simulink model "four_channel_bilateral_teleoperation_architecture_discrete"  (R2021a)
settings: Solver=FixedStepAuto  StartTime=0.0  StopTime=4.0  FixedStep=0.001  RelTol=1e-3
values from neighbouring files (symbols this model uses):
  A = 1    [four_channel_bilateral_teleoperation_architecture_params.m]
  Be = 0    [four_channel_bilateral_teleoperation_architecture_params.m]    (also in params_teleop.m = 100)
  Bh = 70    [four_channel_bilateral_teleoperation_architecture_params.m]    (also in params_teleop.m)
  Bm = 0.8    [four_channel_bilateral_teleoperation_architecture_params.m]    (also in params_teleop.m)
  Bs = 0.8*4    (= 3.2)    [four_channel_bilateral_teleoperation_architecture_params.m]    (also in params_teleop.m)
  Dh = 1000    [four_channel_bilateral_teleoperation_architecture_params.m]
  Dm = 0    [four_channel_bilateral_teleoperation_architecture_params.m]    (also in params_teleop.m)
  Ds = 0    [four_channel_bilateral_teleoperation_architecture_params.m]    (also in params_teleop.m)
  Fc = 1    [four_channel_bilateral_teleoperation_architecture_params.m]
  Fip = 1    [four_channel_bilateral_teleoperation_architecture_params.m]
  Je = 0    [four_channel_bilateral_teleoperation_architecture_params.m]    (also in params_teleop.m)
  Jh = 0.5    [four_channel_bilateral_teleoperation_architecture_params.m]    (also in params_teleop.m)
  Ke = 200    [four_channel_bilateral_teleoperation_architecture_params.m]    (also in params_teleop.m)
  Kh = 2000    [four_channel_bilateral_teleoperation_architecture_params.m]    (also in params_teleop.m)
  Km = 1    [four_channel_bilateral_teleoperation_architecture_params.m]    (also in params_teleop.m)
  Ks = 4    [four_channel_bilateral_teleoperation_architecture_params.m]    (also in params_teleop.m)
  Mm = 0.5    [four_channel_bilateral_teleoperation_architecture_params.m]    (also in params_teleop.m)
  Ms = 2    [four_channel_bilateral_teleoperation_architecture_params.m]    (also in params_teleop.m)
  Ph = 20000    [four_channel_bilateral_teleoperation_architecture_params.m]
  tau = 10000    [four_channel_bilateral_teleoperation_architecture_params.m]
  Ts = 0.001    [four_channel_bilateral_teleoperation_architecture_params.m]
libraries: simulink x7
settings Model: Creator=anuj  LastModifiedBy=antoninoparisi
settings SolverCC: AlgebraicLoopSolver=TrustRegion
settings DebuggingCC: SFMachineParentedDataDiag=warning

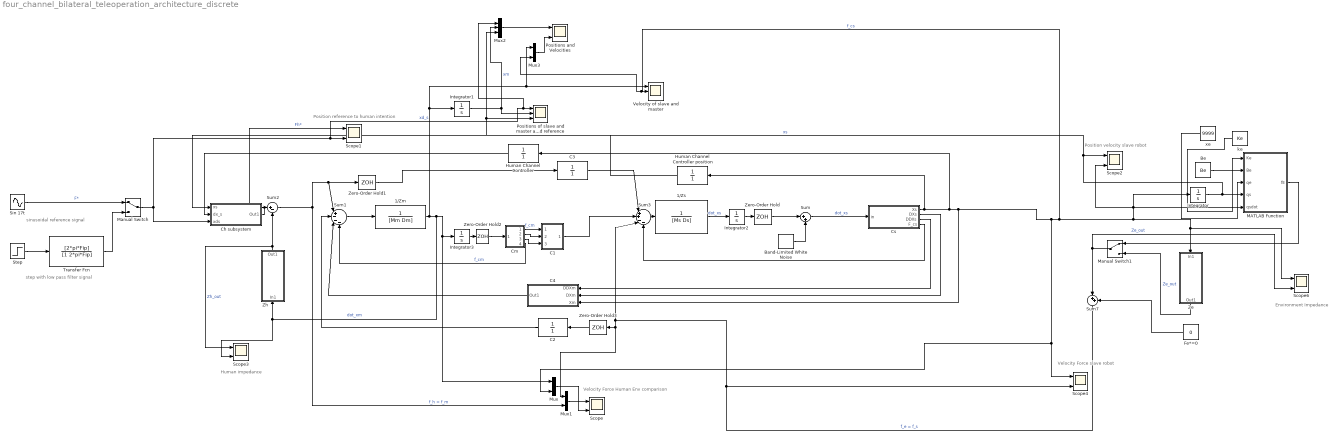
== system four_channel_bilateral_teleoperation_architecture_discrete ==
  note: Environment Impedance
  note: Human impedance
  note: Velocity Force Human Env comparison
  note: Velocity Force slave robot
  note: Position velocity slave robot
  note: sinusoidal reference signal
  note: step with low pass filter signal
  note: Position reference to human intention
  1/Zm : TransferFcn  Denominator=[Mm Dm]
  1/Zs : TransferFcn  Denominator=[Ms Ds]
  Band-Limited White Noise : simulink/Sources/Band-Limited White Noise  Cov=[0.000001]  Ts=Ts  seed=[23341]
  Be : Constant  Value=Be
  C1 : Subsystem
  C2 : TransferFcn  Denominator=[1]
  C3 : TransferFcn  Denominator=[1]
  C4 : Subsystem
  Ch subsystem : Subsystem
  Cm : Subsystem
  Cs : Subsystem
  Fe*=0 : Constant  Value=0
  Human Channel Controller : TransferFcn  Denominator=[1]
  Human Channel Controller position : TransferFcn  Denominator=[1]
  Integrator{,1..3} (4 alike) : Integrator
  MATLAB Function : MATLAB Function  TreatAsAtomicUnit=on
  Manual Switch : ManualSwitch
  Manual Switch1 : ManualSwitch
  Mux : Mux  Inputs=2
  Mux1 : Mux  Inputs=2
  Mux2 : Mux  Inputs=3
  Mux3 : Mux  Inputs=2
  Positions and Velocities : Scope  NumInputPorts=2
  Positions of slave and master and reference : Scope  NumInputPorts=3
  Scope{,1..4,6} (6 alike) : Scope  NumInputPorts=2
  Sin 17t : Sin  Amplitude=A  Frequency=2*pi*Fc  SampleTime=0
  Step : Step  After=A  SampleTime=0
  Sum : Sum  Inputs=|++
  Sum1 : Sum  Inputs=|+---
  Sum2 : Sum  Inputs=|+-
  Sum3 : Sum  Inputs=|++--
  Sum7 : Sum  Inputs=|++
  Transfer Fcn : TransferFcn  Numerator=[2*pi*Fip]  Denominator=[1 2*pi*Fip]
  Velocity of slave and master : Scope  NumInputPorts=3
  Ze : Subsystem
  Zero-Order Hold{,1..3} (4 alike) : ZeroOrderHold  SampleTime=-1
  Zh : Subsystem
  ke : Constant  Value=Ke
  xe : Constant  Value=9999
  wires:
  Mux/1 -> Scope/2
  Mux1/1 -> Scope/1
  Sum2/1 -> Sum1/1, Zero-Order Hold1/1, Mux1/2  "f_h = f_m"
  1/Zm/1 -> Mux3/1, Velocity of slave and master/1, Integrator1/1, Integrator3/1, Mux/1, Zh/1(In1), Scope3/2  "dot_xm"
  Sum1/1 -> 1/Zm/1
  C2/1 -> Sum1/2
  C3/1 -> Sum3/1
  Sum3/1 -> 1/Zs/1
  Fe*=0/1 -> Sum7/2
  Sum7/1 -> Sum3/3, Mux1/1, Zero-Order Hold3/1, Scope4/2  "f_e = f_s"
  C4/1(Out1) -> Sum1/3
  Ch subsystem/1(Out1) -> Scope1/1, Sum2/1  "Fh*"
  Be/1 -> MATLAB Function/2(Be)
  xe/1 -> MATLAB Function/3(qe)
  ke/1 -> MATLAB Function/1(Ke)
  Integrator/1 -> Scope2/1, Positions of slave and master and reference/3, Mux2/3, MATLAB Function/4(qs)  "xs"
  Transfer Fcn/1 -> Manual Switch/2
  Step/1 -> Transfer Fcn/1
  Human Channel Controller/1 -> Ch subsystem/2(dx_s)
  Manual Switch/1 -> Ch subsystem/3(xds), Mux2/1, Positions of slave and master and reference/1, Scope1/2  "xd_s"
  Sin 17t/1 -> Manual Switch/1  "F*"
  C1/1(Out1) -> Sum3/2
  MATLAB Function/1(fE) -> Manual Switch1/1
  Sum/1 -> Cs/1(in)  "dot_xs"
  Manual Switch1/1 -> Sum7/1, Scope6/2  "Ze_out"
  Zh/1(Out1) -> Sum2/2, Scope3/1  "Zh_out"
  Cm/4(F_cm) -> Sum1/4  "f_cm"
  Ze/1(Out1) -> Manual Switch1/2  "Ze_out"
  Integrator1/1 -> Positions of slave and master and reference/2, Mux2/2  "xm"
  Mux2/1 -> Positions and Velocities/1
  Mux3/1 -> Positions and Velocities/2
  1/Zs/1 -> Integrator2/1  "dot_xs"
  Integrator2/1 -> Zero-Order Hold/1
  Zero-Order Hold/1 -> Sum/1
  Zero-Order Hold1/1 -> C3/1
  Cs/1(Xs) -> Human Channel Controller position/1, Human Channel Controller/1, C4/3(Xm), Scope4/1, Mux/2, Mux3/2, Velocity of slave and master/2, MATLAB Function/5(qsdot), Scope2/2, Integrator/1, Scope6/1, Ze/1(In1)  "f_cs"
  Integrator3/1 -> Zero-Order Hold2/1
  Zero-Order Hold2/1 -> Cm/1(In1)
  Cm/1(Xm) -> C1/1(Xm)  "f_cm"
  Cm/2(DXm) -> C1/2(DXm)
  Cm/3(DDXm) -> C1/3(DDXm)
  Cs/3(DDXs) -> C4/1(DDXm)
  Cs/2(DXs) -> C4/2(DXm)
  Cs/4(F_cs) -> Sum3/4
  Band-Limited White Noise/1 -> Sum/2
  Zero-Order Hold3/1 -> C2/1
  Human Channel Controller position/1 -> Ch subsystem/1(xs)

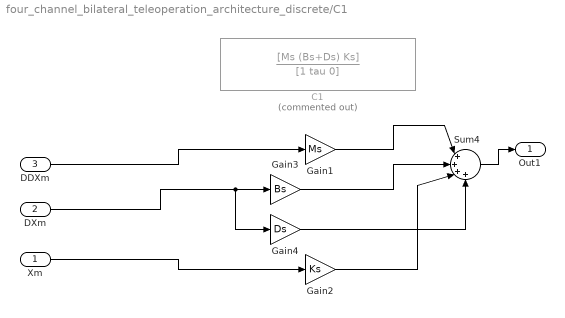
== system four_channel_bilateral_teleoperation_architecture_discrete/C1 ==
  Xm : Inport
  DXm : Inport  Port=2
  DDXm : Inport  Port=3
  C1 : TransferFcn  Commented=on  Numerator=[Ms (Bs+Ds) Ks]  Denominator=[1 tau 0]
  Gain1 : Gain  Gain=Ms
  Gain2 : Gain  Gain=Ks
  Gain3 : Gain  Gain=Bs
  Gain4 : Gain  Gain=Ds
  Sum4 : Sum  Inputs=|++++
  Out1 : Outport
  wires:
  Sum4/1 -> Out1/1
  Gain1/1 -> Sum4/1
  Xm/1 -> Gain2/1
  Gain2/1 -> Sum4/3
  Gain3/1 -> Sum4/2
  Gain4/1 -> Sum4/4
  DDXm/1 -> Gain1/1
  DXm/1 -> Gain4/1, Gain3/1

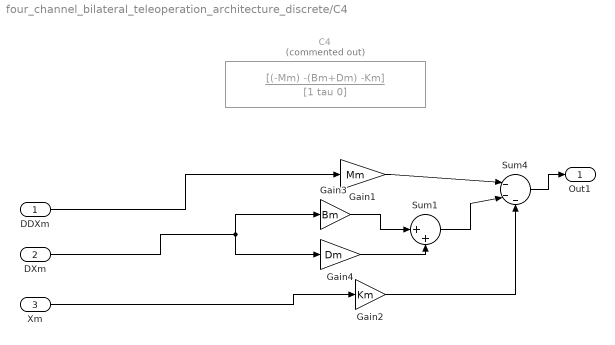
== system four_channel_bilateral_teleoperation_architecture_discrete/C4 ==
  DDXm : Inport
  DXm : Inport  Port=2
  Xm : Inport  Port=3
  C4 : TransferFcn  Commented=on  Numerator=[(-Mm) -(Bm+Dm) -Km]  Denominator=[1 tau 0]
  Gain1 : Gain  Gain=Mm
  Gain2 : Gain  Gain=Km
  Gain3 : Gain  Gain=Bm
  Gain4 : Gain  Gain=Dm
  Sum1 : Sum  Inputs=|++
  Sum4 : Sum  Inputs=|---
  Out1 : Outport
  wires:
  Sum4/1 -> Out1/1
  Gain1/1 -> Sum4/1
  Xm/1 -> Gain2/1
  Gain2/1 -> Sum4/3
  Sum1/1 -> Sum4/2
  Gain4/1 -> Sum1/2
  Gain3/1 -> Sum1/1
  DDXm/1 -> Gain1/1
  DXm/1 -> Gain4/1, Gain3/1

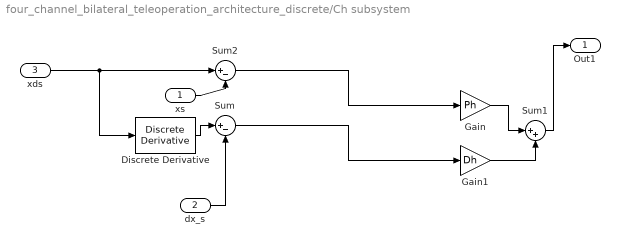
== system four_channel_bilateral_teleoperation_architecture_discrete/Ch subsystem ==
  xs : Inport
  dx_s : Inport  Port=2
  xds : Inport  Port=3
  Discrete Derivative : simulink/Discrete/Discrete Derivative  gainval=1.0  ICPrevScaledInput=0.0  OutMin=[]  OutMax=[]  OutDataType=fixdt(1, 16)  OutScaling=2^-10  DoSatur=off
  Gain : Gain  Gain=Ph
  Gain1 : Gain  Gain=Dh
  Sum : Sum  Inputs=|+-
  Sum1 : Sum  Inputs=|++
  Sum2 : Sum  Inputs=|+-
  Out1 : Outport
  wires:
  Sum1/1 -> Out1/1
  Gain1/1 -> Sum1/2
  Gain/1 -> Sum1/1
  xs/1 -> Sum2/2
  Discrete Derivative/1 -> Sum/1
  Sum/1 -> Gain1/1
  Sum2/1 -> Gain/1
  xds/1 -> Sum2/1, Discrete Derivative/1
  dx_s/1 -> Sum/2

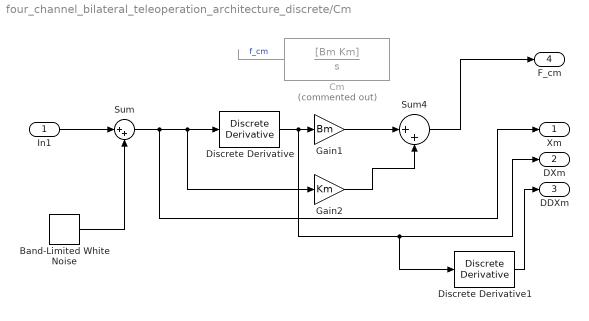
== system four_channel_bilateral_teleoperation_architecture_discrete/Cm ==
  In1 : Inport
  Band-Limited White Noise : simulink/Sources/Band-Limited White Noise  Cov=[0.0000001]  Ts=Ts  seed=[23341]
  Cm : TransferFcn  Commented=on  Numerator=[Bm Km]  Denominator=[1 0]
  Discrete Derivative : simulink/Discrete/Discrete Derivative  gainval=1.0  ICPrevScaledInput=0.0  OutMin=[]  OutMax=[]  OutDataType=fixdt(1, 16)  OutScaling=2^-10  DoSatur=off
  Discrete Derivative1 : simulink/Discrete/Discrete Derivative  gainval=1.0  ICPrevScaledInput=0.0  OutMin=[]  OutMax=[]  OutDataType=fixdt(1, 16)  OutScaling=2^-10  DoSatur=off
  Gain1 : Gain  Gain=Bm
  Gain2 : Gain  Gain=Km
  Sum : Sum  Inputs=|++
  Sum4 : Sum  Inputs=|++
  Xm : Outport
  DXm : Outport  Port=2
  DDXm : Outport  Port=3
  F_cm : Outport  Port=4
  wires:
  Gain1/1 -> Sum4/1
  Gain2/1 -> Sum4/2
  Cm/1 -> ?  "f_cm"
  Discrete Derivative/1 -> Discrete Derivative1/1, DXm/1, Gain1/1
  Discrete Derivative1/1 -> DDXm/1
  Sum4/1 -> F_cm/1
  Band-Limited White Noise/1 -> Sum/2
  In1/1 -> Sum/1
  Sum/1 -> Xm/1, Gain2/1, Discrete Derivative/1

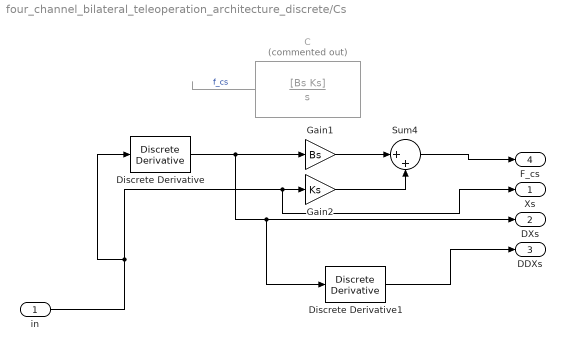
== system four_channel_bilateral_teleoperation_architecture_discrete/Cs ==
  in : Inport
  C : TransferFcn  Commented=on  Numerator=[Bs Ks]  Denominator=[1 0]
  Discrete Derivative : simulink/Discrete/Discrete Derivative  gainval=1.0  ICPrevScaledInput=0.0  OutMin=[]  OutMax=[]  OutDataType=fixdt(1, 16)  OutScaling=2^-10  DoSatur=off
  Discrete Derivative1 : simulink/Discrete/Discrete Derivative  gainval=1.0  ICPrevScaledInput=0.0  OutMin=[]  OutMax=[]  OutDataType=fixdt(1, 16)  OutScaling=2^-10  DoSatur=off
  Gain1 : Gain  Gain=Bs
  Gain2 : Gain  Gain=Ks
  Sum4 : Sum  Inputs=|++
  Xs : Outport
  DXs : Outport  Port=2
  DDXs : Outport  Port=3
  F_cs : Outport  Port=4
  wires:
  Sum4/1 -> F_cs/1
  Gain1/1 -> Sum4/1
  in/1 -> Xs/1, Gain2/1, Discrete Derivative/1
  Gain2/1 -> Sum4/2
  C/1 -> ?  "f_cs"
  Discrete Derivative/1 -> Discrete Derivative1/1, DXs/1, Gain1/1
  Discrete Derivative1/1 -> DDXs/1

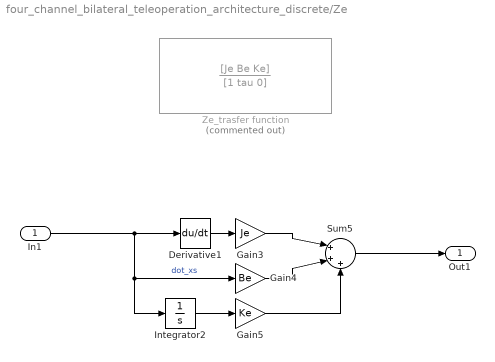
== system four_channel_bilateral_teleoperation_architecture_discrete/Ze ==
  In1 : Inport
  Derivative1 : Derivative
  Gain3 : Gain  Gain=Je
  Gain4 : Gain  Gain=Be
  Gain5 : Gain  Gain=Ke
  Integrator2 : Integrator
  Sum5 : Sum  Inputs=|+++
  Ze_trasfer function : TransferFcn  Commented=on  Numerator=[Je Be Ke]  Denominator=[1 tau 0]
  Out1 : Outport
  wires:
  Gain4/1 -> Sum5/2
  Gain3/1 -> Sum5/1
  Gain5/1 -> Sum5/3
  Sum5/1 -> Out1/1
  Integrator2/1 -> Gain5/1
  In1/1 -> Integrator2/1, Gain4/1, Derivative1/1  "dot_xs"
  Derivative1/1 -> Gain3/1

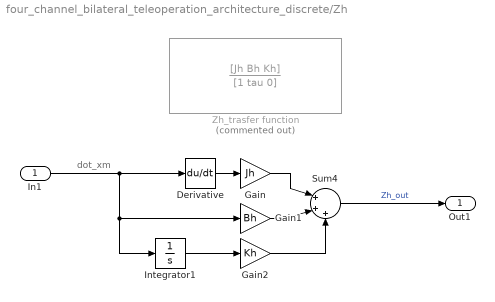
== system four_channel_bilateral_teleoperation_architecture_discrete/Zh ==
  note: dot_xm
  In1 : Inport
  Derivative : Derivative
  Gain : Gain  Gain=Jh
  Gain1 : Gain  Gain=Bh
  Gain2 : Gain  Gain=Kh
  Integrator1 : Integrator
  Sum4 : Sum  Inputs=|+++
  Zh_trasfer function : TransferFcn  Commented=on  Numerator=[Jh Bh Kh]  Denominator=[1 tau 0]
  Out1 : Outport
  wires:
  Derivative/1 -> Gain/1
  Integrator1/1 -> Gain2/1
  Gain2/1 -> Sum4/3
  Gain1/1 -> Sum4/2
  Gain/1 -> Sum4/1
  Sum4/1 -> Out1/1  "Zh_out"
  In1/1 -> Gain1/1, Integrator1/1, Derivative/1

== matlab function four_channel_bilateral_teleoperation_architecture_discrete/MATLAB Function ==
  data: Ke input; fE output; Be input; qe input; qs input; qsdot input
function fE = environment(Ke, Be, qe, qs, qsdot)
    if qs > qe
        fE = Ke * (qs - qe) + Be * qsdot;
    else
        fE = 0;
    end
end
